simulink model "Mag_VarConst"  (R2016b)
settings: Solver=VariableStepAuto  StartTime=0.0  StopTime=10.0  RelTol=1e-3
undefined symbols (not defined in the file or in its folder): Env
settings Model: Creator=rega0051  LastModifiedBy=rega0051
settings DataIOCC: SaveOutput=off  SignalLogging=off  DSMLogging=off  SaveTime=off

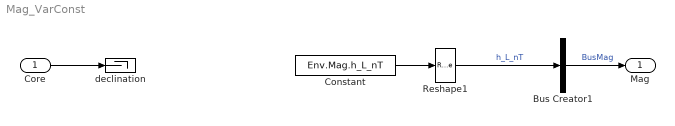
== system Mag_VarConst ==
  Core : Inport  OutDataTypeStr=Bus: BusCore
      settings: AttributesFormatString=%<OutDataTypeStr>
  Bus Creator1 : BusCreator  Inputs=1  OutDataTypeStr=Bus: BusMag
      settings: AttributesFormatString=%<OutDataTypeStr>  InheritFromInputs=off
  Constant : Constant  Value=Env.Mag.h_L_nT
      settings: AttributesFormatString=%<Value>
  Reshape1 : Reshape  OutputDimensionality=Column vector (2-D)  OutputDimensions=[3,1]
  declination : Terminator
  Mag : Outport  OutDataTypeStr=Bus: BusMag
      settings: AttributesFormatString=%<OutDataTypeStr>
  wires:
  Reshape1/1 -> Bus Creator1/1  "h_L_nT"
  Core/1 -> declination/1
  Constant/1 -> Reshape1/1
  Bus Creator1/1 -> Mag/1  "BusMag"
